simulink library "carnot"  (R2018b)
settings: Solver=VariableStepAuto  StartTime=0.0  StopTime=10.0  RelTol=1e-3
undefined symbols (not defined in the file or in its folder): A, A_earth, acol, Acol, ActPower1, ActPower2, ActPower3, Ad, Ad0, Ar, Au, Au0, Azimuth_Angle, B, Bd, Bd0, Br, Bu, Bu0, C, c1, c2, c3, c33, c4, c5, c6, CarnotCallbacks_Density, CarnotCallbacks_Enthalpy, CarnotCallbacks_Enthalpy2Temperature, CarnotCallbacks_Entropy, CarnotCallbacks_Evaporation_Enthalpy, CarnotCallbacks_GlobalMessageLevel, CarnotCallbacks_Grashof, CarnotCallbacks_Heat_Capacity, CarnotCallbacks_Kinematic_Viscosity, CarnotCallbacks_PMV_PPD, CarnotCallbacks_Prandtl, CarnotCallbacks_Saturation_Property, CarnotCallbacks_Saturation_Temperature, CarnotCallbacks_Saturation_Value_Water, CarnotCallbacks_Specific_Volume, CarnotCallbacks_Thermal_Conductivity, CarnotCallbacks_Vapour_Content, CarnotCallbacks_Vapour_Pressure, Cd, Cdl, Cr, Cu, Davies, Dd, DE_TRY2010_04_averageYear, delta_grd, density, DiameterLastPiece, dl, DPConstant, DPLinear, DPQuadratic, Dr ... (+59)
libraries: $bdroot x429, simulink x36, simulink_extras x12
(part 9 of 22)

== system carnot/Source/Energy ==
  Fuel : Subsystem  mask(Configurated Fuels){Temperature=20, Pressure=101300, PathName=fullfile(path_carnot('libsl'), 'Source', 'Energy', 'Fuel', 'parameter_set'), FileName='DefaultFuel_Gas.mat', userPath=off, userParam=off, ft=1, stoichAir=3.5, combustion_enthalpy=[51400000 56900000], Tcondensation=[45 25], massfraction=[0.33 0.67 0 0 0 0], price=1}
      mask prompts: Temperature "Temperature [°C]"; Pressure "pressure [Pa]"; PathName "Path"; FileName "Parameter set"; userPath "Edit path and name of parameter set"; userParam "User defined parameters"; ft "fuel (0=no calculation; 1=gaseous; 2=liquid; 3=solid)"; stoichAir "stoichiometric air demand [kg/kg]"; combustion_enthalpy "heat without/with condensation [J/kg]"; Tcondensation "condensation temperature [°C]"; massfraction "massfraction [H C O S N H2O] [-]"; price "price of fuel per kg [arb. unit]"
      mask help: Fuel source for boiler model (and others). This block uses predefined parameter sets.
      mask init:
      | % callback to set parameters of model
      | [ok, param] = CarnotCallbacks_FuelConf('SetParameters',gcbh,PathName,FileName);
      mask Help: web(fullfile(path_carnot('help'),'Fuel.html'),'-helpbrowser')
      mask TypeOptions Temperature: temperature/Value
      mask TypeOptions Pressure: pressure/Value
      mask Callback userPath: [ok, param] = CarnotCallbacks_FuelConf('UserEdit',gcbh);
      mask Callback userParam: [ok, param] = CarnotCallbacks_FuelConf('UserEdit',gcbh);
      mask TypeOptions ft: fuel_type/Value
      mask TypeOptions stoichAir: airdemand/Value
      mask TypeOptions combustion_enthalpy: enthalpy/Value
      mask TypeOptions Tcondensation: tc/Value
      mask TypeOptions massfraction: mass/Value
      mask TypeOptions price: price/Value
      mask DialogControl Container7 Prompt: Calculation
      mask DialogControl ParameterGroupVar Prompt: Picking a parameter set
      mask DialogControl Control2 Prompt: Carnot public data
      mask DialogControl Control2 Callback: [ok, file] = CarnotCallbacks_FuelConf('GetFilename',gcbh,'public');
      mask DialogControl Control3 Prompt: Carnot internal data
      mask DialogControl Control3 Callback: [ok, file] = CarnotCallbacks_FuelConf('GetFilename',gcbh,'internal');
      mask DialogControl Control4 Prompt: Selected path
      mask DialogControl Control4 Callback: [ok, file] = CarnotCallbacks_FuelConf('GetFilename',gcbh,'selected');
      mask DialogControl Container5 Prompt: Properties
      mask DialogControl Container6 Prompt: Eco
      mask DialogControl Control6 Prompt: Save in Carnot internal data
      mask DialogControl Control6 Callback: [ok, param] = CarnotCallbacks_FuelConf('SaveFilename',gcbh,'internal','FUEL');
      mask DialogControl Control7 Prompt: Save in selected path
      mask DialogControl Control7 Callback: [ok, param] = CarnotCallbacks_FuelConf('SaveFilename',gcbh,'selected','FUEL');
      mask Display:
      | % user defined picture file
      | picfile = fullfile(path_carnot('intlibsl'), ...
      |     'Source','Energy','Fuel','parameter_set', ...
      |     'Fuel_CONF.jpg');
      | 
      | pic = false;
      | 
      | % show internal picture if defined
      | if ~BlockIsInCarnotLibrary    % if not located in library any more
      |     if exist(picfile)
      |         image(imread(picfile), [0.1, 0, 0.8, 1])
      |         set_param(gcb, 'BackgroundColor', 'White')
      |         pic = true;
      |     end
      | end
      | 
      | if ~pic   % show public picture
      |     set_param(gcb, 'BackgroundColor', 'Magenta')
      |     plot(0,0,1,1, ...
      |         [90,67,84,63,80,60,70,90,80,80,70,20,10,10,20,60]/120, ...
      |         [70,87,64,83,60,80,90,70,60,10,0,0,10,70,80,80]/100, ...
      |         [30,60,60,40,40,50,50,40,40,30,30]/120, ...
      |         [60,60,50,50,40,40,30,30,10,10,60]/100)
      | end

== system carnot/Source/Heat_Exchanger ==
  Floorheating_TABS : Subsystem  mask(FBH-TABS){d=0.08, d1=0.04, d_pipe=0.016, dr=0.002, dx=0.1, l=700, lambda_r=0.35, lambda_b=1.4}
      mask prompts: d "thickness of active layer [m]"; d1 "depth of pipes in active layer [m]"; d_pipe "outer diameter of pipes [m]"; dr "wall thickness of pipe [m]"; dx "distance between center of pipes [m]"; l "length of pipe [m]"; lambda_r "conductivity of pipe [W/(m*K)]"; lambda_b "conductivity of layer material [W/(m*K)]"
      mask help:
      | calculates the heating/cooling power from pipes
      | in a floor heating system or a thermally active building component
      | to the active layer in the building element (wall, floor, ceiling)
      | according to the model of M.Koschenz & B.Lehmann, EMPA-CH, 2000
      mask Help: web(fullfile(path_carnot('help'),'FHB_TABS.html'),'-helpbrowser')
  HeatExchanger : Subsystem  mask(heat exchanger){flowtype=1, ua0=2000, uahot=[0.1 0], uacold=[0.1 0], ualoss=1, cap=2*4182, linh=20, quah=10, linc=20, quac=10, t0=20}
      mask prompts: flowtype "type of flow (0 = parallel, 0.5 = cross, 1 = counter)"; ua0 "constant heat transfer ua0 [W/K]"; uahot "[mdot_nom_pri [kg/s],  ua_exp_pri]"; uacold "[mdot_nom_sec [kg/s],  ua_exp_sec]"; ualoss "heat losses to ambient [W/K]"; cap "capacity [J/K]"; linh "Source: pressure drop linear in massflow [Pa*s/kg]"; quah "Source: pressure drop quadratic in massflow [Pa*s²/kg²]"; linc "Load: pressure drop linear in massflow [Pa*s/kg]"; quac "Load: pressure drop quadratic in massflow [Pa*s²/kg²]"; t0 "initial temperature [degree centigrade]"
      mask help:
      | Model of a heat exchanger using the NTU approach
      | The heat transfer is:
      | ua = ua0 * ( (mdot_pri/mdot_nom_pri)^ua_exp_pri
      |      + (mdot_sec/mdot_nom_sec)^ua_exp_sec )/2
      mask Help: web(fullfile(path_carnot('help'),'HeatExchanger.html'),'-helpbrowser')
      mask DialogControl ParameterTabVar0 Prompt: Thermal
      mask DialogControl ParameterTabVar01 Prompt: Hydraulic
      mask DialogControl ParameterTabVar012 Prompt: Calculation
      mask Display: plot(-10,20,115,100,[40,70,70,40,40],[40 40 70 70 40],[55 55 62 48 55 55],[25 40 55 55 70 85],[30 40],[55 55],[70 80],[55 55])
  Radiator : Subsystem  mask(Radiator){pnom=500, dtnom=49.83, expo=1.3, mcap=5*4182, tini=20, lin=10, qua=10}
      mask prompts: pnom "Qdot_nom: nominal power in W"; dtnom "Tdiff_nom: nominal temperature difference in K"; expo "radiator exponent (> 0)"; mcap "mass * capacity per unit in J/K"; tini "Initial temperature in °C"; lin "l : linear pressure drop Pa/(kg/s)"; qua "q : quadratic pressure drop Pa/(kg/s)²"
      mask help:
      | Calculates the power of a radiator according to the nominal power the and the temperature difference (EN 442).
      | Qdot = Qdot_nom * (Tdiff/Tdiff_nom)^exponent
      | Tdiff_nom for EN 442 test is 49.83 K
      | The thermal capacity of the radiator is modeled by a 1-node capacity.
      | mcp*dTnode/dt = mdot*cp*(Tin-Tnode)-Qdot
      | In difference to EN 442 the outlet temperature is Tnode. Tnode is not calculated as average temperature of inlet and outlet.
      | A quadratic pressure drop is applied to the fluid flow.
      mask Help: web(['file:///' fullfile(path_carnot('help'),'Radiator.html')],'-helpbrowser')
      mask TypeOptions pnom: Radiator_basic/pnomEN
      mask TypeOptions dtnom: Radiator_basic/dtnomEN
      mask TypeOptions expo: Radiator_basic/expo
      mask TypeOptions mcap: Radiator_basic/mcp
      mask TypeOptions tini: Radiator_basic/tini
      mask TypeOptions lin: pressdrop_fix_THB/lin
      mask TypeOptions qua: pressdrop_fix_THB/qua
      mask DialogControl ParameterTabVar0 Prompt: Thermal
      mask DialogControl ParameterTabVar01 Prompt: Hydraulic
      mask Display: plot(-20,0,120,90,[20 90 90 20 20],[20 20 70 70 20],[30 30],[25 65],[40 40],[25 65],[50 50],[25 65],[60 60],[25 65],[70 70],[25 65],[80 80],[25 65],[15 20],[25 25],[15 20],[65 65])
  Radiator_AIV : Subsystem  mask(radiator){pnom=500, dtnom=40, expo=1.3, mcap=5*4182, ra=0.47, tini=20, lin=10, qua=10}
      mask prompts: pnom "nominal power per unit in W"; dtnom "nominal temperature difference in K"; expo "radiator exponent (> 0)"; mcap "mass * capacity per unit in J/K"; ra "radiative part of heat transfer (0..1)"; tini "initial temperature in degree Celsius"; lin "linear pressure drop dependace of massflow in Pa*s/kg"; qua "quadratic pressure drop dependace of massflow in Pa*s²/kg²"
      mask help: Calculates the power of a radiator according to the nominal power the and the temperaure difference.
      mask init:
      | ra = max(0, min(1, ra));
      | co = 1-ra;
      mask Help: web(['file:///' fullfile(path_carnot('help'),'Radiator.html')],'-helpbrowser')
      mask DialogControl ParameterTabVar0 Prompt: Thermal
      mask DialogControl ParameterTabVar01 Prompt: Hydraulic
      mask Display: plot(-20,0,120,90,[20 90 90 20 20],[20 20 70 70 20],[30 30],[25 65],[40 40],[25 65],[50 50],[25 65],[60 60],[25 65],[70 70],[25 65],[80 80],[25 65],[15 20],[25 25],[15 20],[65 65])
  THB_P_adapter : Subsystem  mask(ACTIVE COMPONENT){mass=1, ua=800*5*5/0.2*0.022*3.1415, t0=20}
      mask prompts: mass "MASS of fluid in heating element >0, kg"; ua "HEAT TRANSFER of fluid <-> wall >0, W/K"; t0 "start temperature in °C"
      mask help:
      | Adapter between active components and house-model.
      | Transformation from heat flow - defined by the thermo-hydraulic vector THB - to a power entering the block "active wall", "active ceiling", "active floor" or "flat radiator".
      | P  : "electric" power flowing into active layer of wall, W
      | T(P)  : temperature of active layer, °C
      | THB_in  : hydraulic vector input
      | THB_out : hydraulic vector output
      mask init:
      | % mass = str2num(mass);
      | % if length(mass)~=1 error(['PARAMETERS block "' path2block '" : "MASS ..." must have only 1 entry !']); end;
      | % if (mass<=0) error(['PARAMETERS block "' path2block '" : "MASS ..." must be >0 !']); end;
      | % 
      | % ua = str2num(ua);
      | % if length(ua)~=1 error(['PARAMETERS block "' path2block '" : "HEAT TRANSFER ..." must have only 1 entry !']); end;
      | % if (ua<=0) error(['PARAMETERS block "' path2block '" : "HEAT TRANSFER ..." must be >0 !']); end;
      mask Help: web(fullfile(path_carnot('help'),'THB_P_adapter.html'),'-helpbrowser')
  VDIHeatExchanger : Subsystem  mask(VDI heat exchanger){t0=20, PathName=fullfile(path_carnot('intlibsl'), 'Source', 'Heat_Exchanger', 'VDIHeatExchanger', 'parameter_set'), FileName='<user defined>', userPath=off, userParam=off, flowtype=1, a=0, b=0, c=0, d=0, ua0=2000, uahot=[0.04 0], uacold=[0.04 0], ualoss=3, cap=10e3, linh=20, quah=10, linc=20, quac=10}
      mask prompts: t0 "initial temperature [degree centigrade]"; PathName "Path"; FileName "Parameter set"; userPath "Edit path and name of parameter set"; userParam "User defined parameters"; flowtype "type of flow (0 = parallel, 0.5 = cross, 1 = counter)"; d "d (0.5 for symetric heat exchangers)"; ua0 "constant heat transfer ua0 [W/K]"; uahot "[mdot_nom_hot [kg/s] (>0) ,  ua_exp_hot (>=0)]"; uacold "[mdot_nom_cold [kg/s] (>0) ,  ua_exp_cold (>=0)]"; ualoss "heat losses to ambient [W/K]"; cap "capacity [J/K]"; linh "Source: pressure drop linear in massflow [Pa*s/kg]"; quah "Source: pressure drop quadratic in massflow [Pa*s²/kg²]"; linc "Load: pressure drop linear in massflow [Pa*s/kg]"; quac "Load: pressure drop quadratic in massflow [Pa*s²/kg²]"
      mask help:
      | Calculates the output THB of the hot and cold fluid of a heat exchanger.
      | The heat transfer is:
      | 	ua = ua0 * ( (mdot_hot/mdot_nom_hot)^ua_exp_hot
      |      	+ (mdot_cold/mdot_nom_cold)^ua_exp_cold )/2
      mask init:
      | flowtype = max(0, min(flowtype, 1));
      | linh = max(linh,0);
      | linc = max(linc,0);
      | quah = max(quah,0);
      | quac = max(quac,0);
      | uahot(1) = max(uahot(1), 1e-4);
      | uahot(2) = max(uahot(2), 0);
      | uacold(1) = max(uacold(1), 1e-4);
      | uacold(2) = max(uacold(2), 0);
      | cap = max(cap, 0.01);
      mask Help: web(fullfile(path_carnot('inthelp'),'VDIHeatExchanger.html'),'-helpbrowser')
      mask Callback userPath: [ok, param] = CarnotCallbacks_VDIHeatexchangerConf('UserEdit',gcbh);
      mask Callback userParam: [ok, param] = CarnotCallbacks_VDIHeatexchangerConf('UserEdit',gcbh);
      mask DialogControl Container14 Prompt: Calculation
      mask DialogControl ParameterGroupVar Prompt: Picking a parameter set
      mask DialogControl Control2 Prompt: Carnot public data
      mask DialogControl Control2 Callback: [ok, file] = CarnotCallbacks_VDIHeatexchangerConf('GetFilename',gcbh, 'public');
      mask DialogControl Control3 Prompt: Carnot internal data
      mask DialogControl Control3 Callback: [ok, file] = CarnotCallbacks_VDIHeatexchangerConf('GetFilename',gcbh, 'internal');
      mask DialogControl Control4 Prompt: Selected path
      mask DialogControl Control4 Callback: [ok, file] = CarnotCallbacks_VDIHeatexchangerConf('GetFilename',gcbh, 'selected');
      mask DialogControl ParameterTabVar0 Prompt: Thermal
      mask DialogControl Container9 Prompt: parameters for correction factor
      mask DialogControl ParameterTabVar01 Prompt: Hydraulic
      mask DialogControl Control5 Prompt: Save in Carnot internal data
      mask DialogControl Control5 Callback: [ok, param] = CarnotCallbacks_VDIHeatexchangerConf('SaveFilename',gcbh, 'internal','USTC');
      mask DialogControl Control6 Prompt: Save in selected path
      mask DialogControl Control6 Callback: [ok, param] = CarnotCallbacks_VDIHeatexchangerConf('SaveFilename',gcbh, 'selected','USTC');
      mask Display:
      | plot(-10,15,120,100,[40,70,70,40,40],[40 40 70 70 40],[55 55 62 48 55 55],[25 40 55 55 70 85],[30 40],[55 55],[70 80],[55 55])
      | disp('VDI')
      | port_label('input',1,'Ta')
      | port_label('input',2,'THBpri')
      | port_label('input',3,'THBsec')
      | port_label('output',1,'THBpri')
      | port_label('output',2,'THBsec')

== system carnot/Source/Heat_Pump ==
  Ground_Source_Heat_Exchanger : Subsystem  mask(ground source heat exchanger){Jahresmitteltemp_C=10, TGrad=0.025, lambdaErde=2.5, cpErde=1000, rhoErde=2200, lambdaFill=0.81, cpFill=3040, rhoFill=1180, lambda_Sondenrohr=0.48, dTdesign=5, Sondenlaenge=100, B_sondenabstand=10, Sondendurchmesser=0.026+2*0.003, Bohrdurchmesser=0.12, Bu_param=0.06, Wanddicke_Sondenrohr=0.003, SondenFall=5x10 probes B/H = 0.1, DimVert=5, DimRad=10, Gitterfaktor=2.5, LastYear=1, show=off}
      mask prompts: Jahresmitteltemp_C "Average annual outdoor temperature  in °C"; TGrad "Temperature gradient in K/m, typical 0.025..0.04"; lambdaErde "Thermal conductivity ground in W/m/K"; cpErde "Heat capacity of the ground in J/kg/K"; rhoErde "Denstiy of the ground in kg/m³"; lambdaFill "Thermal conductivity filling in W/m/K"; cpFill "Heat capacity of the filling in J/kg/K"; rhoFill "Denstiy of the filling in kg/m³"; lambda_Sondenrohr "Thermal conductivity of pipe material  in W/m/K"; dTdesign "Design temperature difference inlet-outlet in K"; Sondenlaenge "H: Length of earth probe in m"; B_sondenabstand "B: Probe distance in m (= calculation diameter for single probe)"; Sondendurchmesser "Diameter of tube in m"; Bohrdurchmesser "Diameter of drilled hole in m"; Bu_param "Shank spacing in m (must be < borehole diameter)"; Wanddicke_Sondenrohr "Thickness of pipe wall in m"; SondenFall "Field geometry"; DimVert "No. of vertical nodes (typical 5, minimum 2)"; DimRad "No. of horizontal (radial) nodes (typical 10, minimum 3)"; Gitterfaktor "grid factor (typical 2.5, must be > 1)"; LastYear "Year of ground temperature pre-calculation (steady state = 50)"; show "Display start conditions"
      mask help: The CARNOT EWS model is a transient model for dynamic simulation of borehole heat exchangers or so-called vertical ground heat exchangers. The model is based on the equations described by [Huber] and has been implemented using the state space model of Matlab/Simulink [Bianchi]. See <Help> for literature.
      mask init:
      | startfall = 2;
      | DimAxi = max(DimVert*2,4);
      | DimRad = max(DimRad,3);
      | 
      | [Ad,Bd,Cd,Dd, Au,Bu,Cu,Du, Ad0,Bd0, Au0,Bu0, ...
      |     Ar,Br,Cr,Dr, Cdl, c1, c3, c31, c33, c4, c41, c5, c6, ...
      |     L1, L2, L10, L20, dl, Rechenradius, np, ...
      |     Tearth_anf, T_null, teta_fluid_ini, Tdown_0, Tup_0, ...
      |     Ts_Trichter, t_Trichter, r_Trichter, gfunction, t_start ...
      |     ] = ...
      |     CarnotCallbacks_EWS(startfall, LastYear, dTdesign, ...
      |     SondenFall, B_sondenabstand, Sondenlaenge, Sondendurchmesser, ...
      |     Bohrdurchmesser, Bu_param, Wanddicke_Sondenrohr, ...
      |     Jahresmitteltemp_C, TGrad, ...
      |     lambdaErde, rhoErde, cpErde, ...
      |     lambdaFill, cpFill, rhoFill, lambda_Sondenrohr, ...
      |     DimAxi, DimRad, Gitterfaktor, show);
      mask Help: web(fullfile(path_carnot('help'),'Ground_Source_Heat_Exchanger.html'),'-helpbrowser')
      mask TypeOptions SondenFall: 1 probe | 2 probes B/H = 0.1 | 2 probes B/H = 0.05 | 3x6 probes B/H = 0.1 | 5x10 probes B/H = 0.1
      mask DialogControl ParameterTabVar0 Prompt: Thermal
      mask DialogControl ParameterTabVar01 Prompt: Geometry
      mask DialogControl ParameterTabVar012 Prompt: Calculation
      mask Display:
      | plot(0,10,100,90,[70,30],[80,80], ...
      |     [35,35,43,43,47,52,57,57,66,66,60,60,54,46,40,40,35], ...
      |     [84,87,87,20,13,13,21,87,87,84,84,20,10,10,20,84,84])
  HeatPump : Subsystem  mask(Heat Pump CONF){PathName=fullfile(path_carnot('libsl'), 'Source','Heat_Pump','HeatPump','parameter_set'), FileName='<user defined>', userPath=off, userParam=off, K=[300 -60 12250 -6.666666 60 -5.1315833e-05 306.66666 -115 12225], caph=32000, capc=32000, UA=6, relQdotMin=1, linc=10, quac=100, linh=10, quah=100}
      mask prompts: PathName "Path"; FileName "Parameter set"; userPath "Edit path and name of parameter set"; userParam "User defined parameters"; K "Parameters K (see also HP_param.m)"; caph "thermal capacity hot loop [J/K]"; capc "thermal capacity cold loop [J/K]"; UA "heat loss coefficient [W/K]"; relQdotMin "Minimum control signal for "on" (0...1)"; linc "cold side: linear pressure drop Pa/(kg/s)"; quac "cold side: quadratic pressure drop Pa/(kg/s)²"; linh "hot side : linear pressure drop Pa/(kg/s)"; quah "hot side: quadratic pressure drop Pa/(kg/s)²"
      mask help:
      | Configurated heat pump model, variables are defined in a mat-file (for example in "DefaultHeatPump.mat"). The linearized heat pump model uses measured data (e.g. EN 14511).
      | This block uses predefined parameter sets.
      | -   heating_power = K1 * Tprimary + K2 * Tsecondary + K3
      | -   electric_power = K4 * Tprimary + K5 * Tsecondary + K6
      | -   absorbing_power = K7 * Tprimary + K8 * Tsecondary + K9
      mask init:
      | % callback to set parameters of model
      | [ok, param] = CarnotCallbacks_HeatPump('SetParameters',gcbh,PathName,FileName);
      mask Help: web(fullfile(path_carnot('help'),'heatpump.html'),'-helpbrowser')
      mask Callback userPath: [ok, param] = CarnotCallbacks_HeatPump('UserEdit',gcbh);
      mask Callback userParam: [ok, param] = CarnotCallbacks_HeatPump('UserEdit',gcbh);
      mask TypeOptions K: HeatPump_basic/K
      mask TypeOptions caph: HeatPump_basic/caph
      mask TypeOptions capc: HeatPump_basic/capc
      mask TypeOptions UA: HeatPump_basic/UA
      mask TypeOptions relQdotMin: Switch/Threshold
      mask TypeOptions linc: Pressure_Drop_Cold/lin
      mask TypeOptions quac: Pressure_Drop_Cold/qua
      mask TypeOptions linh: Pressure_Drop_Hot/lin
      mask TypeOptions quah: Pressure_Drop_Hot/qua
      mask DialogControl Control1 Prompt: Carnot public data
      mask DialogControl Control1 Callback: [ok, file] = CarnotCallbacks_HeatPump('GetFilename',gcbh,'public');
      mask DialogControl Control3 Prompt: Carnot internal data
      mask DialogControl Control3 Callback: [ok, file] = CarnotCallbacks_HeatPump('GetFilename',gcbh,'internal');
      mask DialogControl Control4 Prompt: Selected path
      mask DialogControl Control4 Callback: [ok, file] = CarnotCallbacks_HeatPump('GetFilename',gcbh,'selected');
      mask DialogControl Container6 Prompt: HP Characteristic
      mask DialogControl Container7 Prompt: Hydraulic
      mask DialogControl Control5 Prompt: Save in Carnot internal data
      mask DialogControl Control5 Callback: [ok, param] = CarnotCallbacks_HeatPump('SaveFilename',gcbh,'internal','HP');
      mask DialogControl Control6 Prompt: Save in selected path
      mask DialogControl Control6 Callback: [ok, param] = CarnotCallbacks_HeatPump('SaveFilename',gcbh,'selected','HP');
      mask Display:
      | % user defined picture file
      | picfile = fullfile(path_carnot('intlibsl'), ...
      |     'Source','Heat_Pump','HeatPump','parameter_set', ...
      |     'HeatPump_CONF.jpg');
      | 
      | pic = false;
      | 
      | % show internal picture if defined
      | if ~BlockIsInCarnotLibrary    % if not located in library any more
      |     if exist(picfile)
      |         image(imread(picfile), [0.1, 0, 0.8, 1])
      |         set_param(gcb, 'BackgroundColor', 'White')
      |         pic = true;
      |     end
      | end
      | 
      | if ~pic   % show public picture
      |     set_param(gcb, 'BackgroundColor', 'Red')
      |     plot([10,20,40,60,80,90,90,80,60,40,20,10,10]/100, ...
      |         [60,80,90,90,80,60,40,20,10,10,20,40,60]/100,[40,20]/100,...
      |         [90,20]/100,[60,80]/100,[90,20]/100,[50,50]/100, ...
      |         [30,50]/100,[60,40]/100,[40,40]/100,...
      |         [57,43]/100,[33,46]/100,[44,57]/100,[34,46]/100)
      | end

== system carnot/Source/Simple ==
  Constant_EB : Subsystem  mask(constant EB){eID=Power only, f=50, v1=230, p1=0, pf1=1, v2=230, p2=0, pf2=1, v3=230, p3=0, pf3=1}
      mask prompts: eID "ID"; f "frequency [Hz]"; v1 "voltage to ground [V]"; p1 "active  power [W]"; pf1 "power factor[-]"; v2 "voltage to ground [V]"; p2 "active  power [W]"; pf2 "power factor[-]"; v3 "voltage to ground [V]"; p3 "active  power [W]"; pf3 "power factor[-]"
      mask help: Create a constant Electric-Bus.
      mask Help: web(fullfile(path_carnot('help'),'Constant_EB.html'),'-helpbrowser')
      mask TypeOptions eID: basic_EB/eID
      mask TypeOptions f: basic_EB/f
      mask TypeOptions v1: basic_EB/v1
      mask TypeOptions p1: basic_EB/p1
      mask TypeOptions pf1: basic_EB/pf1
      mask TypeOptions v2: basic_EB/v2
      mask TypeOptions p2: basic_EB/p2
      mask TypeOptions pf2: basic_EB/pf2
      mask TypeOptions v3: basic_EB/v3
      mask TypeOptions p3: basic_EB/p3
      mask TypeOptions pf3: basic_EB/pf3
      mask DialogControl ParameterTabVar012_copy Prompt: Common
      mask DialogControl ParameterTabVar0 Prompt: Line 1
      mask DialogControl ParameterTabVar01 Prompt: Line2
      mask DialogControl ParameterTabVar012 Prompt: Line3
  Constant_THB : Subsystem  mask(constant THB){t=20, mdot=0, p=1e5, mID=No Pressure Drop, fluid=Water, mix=0, mix2=0, mix3=0, dia=0.02, hgt=0}
      mask prompts: t "temperature [degree centigrade]"; mdot "massflow [kg/s]"; p "pressure [Pa]"; mID "ID (for pressure drop calculation)"; mix "fluid mixture [0..1]"; mix2 "fluid mixture 2 [0..1]"; mix3 "fluid mixture 3 [0..1]"; dia "diameter [m]"; hgt "Static height in m"
      mask help: Create a constant Thermo-Hydraulic-Bus.
      mask Help: web(fullfile(path_carnot('help'),'constant_THB.html'),'-helpbrowser')
      mask TypeOptions t: basic_THB/t
      mask TypeOptions mdot: basic_THB/mdot
      mask TypeOptions p: basic_THB/p
      mask TypeOptions mID: basic_THB/ID
      mask TypeOptions fluid: basic_THB/fluid
      mask TypeOptions mix: basic_THB/mix
      mask TypeOptions mix2: basic_THB/mix2
      mask TypeOptions mix3: basic_THB/mix3
      mask TypeOptions dia: basic_THB/dia
      mask TypeOptions hgt: basic_THB/hgt
      mask DialogControl ParameterTabVar0 Prompt: Hydraulic
      mask DialogControl ParameterTabVar01 Prompt: Fluid
      mask DialogControl ParameterTabVar012 Prompt: Geometry
  EB_set_power : Subsystem  mask(EB_set_power){}
      mask help: Set the active power in the electric bus.
      mask Help: web(['file:///' fullfile(path_carnot('help'),'EB_set_power.html')],'-helpbrowser')
  EB_set_voltage : Subsystem  mask(EB_set_voltage){}
      mask help: Set the voltages in the electric bus.
      mask Help: web(['file:///' fullfile(path_carnot('help'),'EB_set_voltage.html')],'-helpbrowser')
  THB_fixed_T : Subsystem  InitFcn=load('THB.mat');  mask(set temperature in THB){t=60}
      mask prompts: t "temperature in degree Celsuis"
      mask help: Set a constant temperature in the thermo-hydraulic bus.
      mask Help: web(fullfile(path_carnot('help'),'THB_fixed_T.html'),'-helpbrowser')
  THB_fixed_mdot : Subsystem  InitFcn=load('THB.mat');  mask(set masssflow in THB){m=10/60}
      mask prompts: m "massflow in kg/s"
      mask help: Set a constant massflow in the thermo-hydraulic vector.
      mask Help: web(fullfile(path_carnot('help'),'THB_fixed_mdot.html'),'-helpbrowser')
  THB_set_T : Subsystem  InitFcn=load('THB.mat');  mask(set temperature in THB){}
      mask help: Set a variable temperature in the thermo-hydraulic bus.
      mask Help: web(['file:///' fullfile(path_carnot('help'),'THB_set_T.html')],'-helpbrowser')
  THB_set_mdot : Subsystem  InitFcn=load('THB.mat');  mask(set massflow in THB){}
      mask help: Set the mass flow rate in the thermo-hydraulic bus.
      mask Help: web(['file:///' fullfile(path_carnot('help'),'THB_set_mdot.html')],'-helpbrowser')
  create_EB : Subsystem  mask(create EB){eID=Power only, f=50, pf1=1, pf2=1, pf3=1}
      mask prompts: eID "ID for electric calculation"; f "frequency [Hz]"; pf1 "power factor line 1 [1]"; pf2 "power factor line 2 [1]"; pf3 "power factor line 3 [1]"
      mask help: Block to create an EB with the variable inputs ActivePower and Voltage. The other values can be set as constants in the mask.
      mask Help: web(fullfile(path_carnot('help'),'create_EB.html'),'-helpbrowser')
      mask TypeOptions eID: basic_create_EB/eID
      mask TypeOptions f: basic_create_EB/f
      mask TypeOptions pf1: basic_create_EB/pf1
      mask TypeOptions pf2: basic_create_EB/pf2
      mask TypeOptions pf3: basic_create_EB/pf3
  create_THB : Subsystem  mask(create THB){p=1e5, fluid=Water, mix=0, mix2=0, mix3=0, dia=0, hgt=0, mID=No Pressure Drop}
      mask prompts: p "pressure [Pa]"; mix "fluid mixture [0..1]"; mix2 "fluid mixture 2 [0..1]"; mix3 "fluid mixture 3 [0..1]"; dia "diameter [m]"; hgt "Geodetic height in m"; mID "ID (for pressure drop calculation)"
      mask help: Block to create a THB with the variable input T and mdot. The other value can be set as constants in the mask.
      mask init:
      | mix = min(1, max(0, mix));
      | dia = max(dia, 0.001);
      | ID = (mID-1)*10000+1;
      mask Help: web(fullfile(path_carnot('help'),'createTHB.html'),'-helpbrowser')
      mask TypeOptions p: basic_create_THB/p
      mask TypeOptions fluid: basic_create_THB/fluid
      mask TypeOptions mix: basic_create_THB/mix
      mask TypeOptions mix2: basic_create_THB/mix2
      mask TypeOptions mix3: basic_create_THB/mix3
      mask TypeOptions dia: basic_create_THB/dia
      mask TypeOptions hgt: basic_create_THB/hgt
      mask TypeOptions mID: basic_create_THB/mID
